simulink model "ComplexPhaseDetectorDual"  (R2016a)
settings: Solver=VariableStepAuto  StartTime=0.0  StopTime=.05  RelTol=1e-6
PreLoadFcn:
  | Bits = 4
  | Ts=2*3/280e6
  | dBRange=11
  | maxNumErrs=500
  | maxNumBits=1e6
  | AM_Gain=AM_GainDiff;
  | AGC_Gain=AGC_GainCalc;
  | load('IIR_Coeffs.mat');
InitFcn:
  | Br= 1/(10*Ts)
  | FreqOffset=00
  | Mode=2
  | BitsPer=[2,2,1,1]
  | EbNo=50
  | N=6
undefined symbols (not defined in the file or in its folder): designMultirateFIR, DiscIntNeverNeededParam
libraries: xbsIndex_r4 x1085, commfilt2 x12, commsink2 x6, dspsigops x5, dspmlti4 x2, commrfcorlib x2, commchan3 x2, dspfdesign x2, dspstat3 x2, commdigbbndpm3 x1, commrandsrc3 x1
(part 1 of 13)
settings Model: Creator=frank.ziegler  LastModifiedBy=frank
settings DebuggingCC: ConsistencyChecking=warning  ArrayBoundsChecking=error  UniqueDataStoreMsg=error

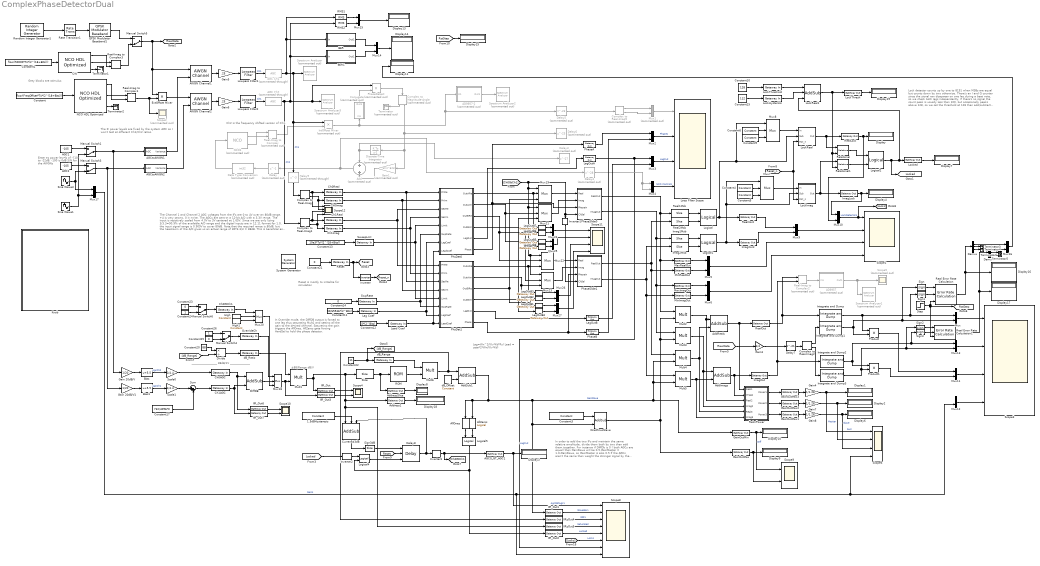
== system ComplexPhaseDetectorDual ==
  note: Lag=Wn^2/(Kv*Kd*Fs)
      | Lead = zeta*2*Wn/(Kv*Kd)
  note: Lock detector counts up by one to 8191 when MSBs are equal but counts down by two otherwise. There's an I and Q counter since the signal can disappear on one leg during a beat note, so we check both legs independently. If there's no signal the count peak is usually less than 100, but occasionally peaks above 128, so we set the threshold at 128 then add/subtract 112 of hysterisis such that both signals have to drop below 16 to loose lock, then either rise above 240. This gives a strong confidence to the lock and allows the 8192 a long time (76uS) to count down to 256 during a fade.
      | Note, the higher the beat note in the IF, the more false negative at high noise levels. At 800Hz I've seen an error every 10 seconds or so.
  note: Reset is mostly to initialize for simulation
  note: Enter as power levels of -110 to -22dB.
      | -100 is 0dB S/N for the AWGNs
  note: The IF power levels are fixed by the system AGC so I won't test at different Ch1/Ch2 ratios.
  note: Ch2 is the frequency shifted version of Ch1.
  note: The Channel 1 and Channel 2 AGC voltages from the IFs are 0 to 4V over an 80dB range. +4 is very strong, 0 is noise. The AGCs are sent to a 12-bit A/D with a 3.3V range. The input is resistively scaled from 4.0V to 3V centered at 1.65V. Since we are only using 3/3.3=90.9% of the available A/D range and the digital inputs are in 12.11 format for 1.0, the input signal range is 0.909V to cover 80dB.
      | Note that the required range is 80dB, but the headroom of the A/D gives us an actual range of 80*3.3/3 = 88dB. This is beneficial as shown below.
      | We take the difference in AGC voltage between the two channels to define the weighting system based on the stronger signal. If we take the differential and multiply by 8 with saturation this effectively gives us a ± 11dB differential maximum. We can use this to limit the range the combiner attempts to work over since combining is only useful over a 10dB range. The nature of the saturation forces a "Best Source Select" function automatically. We take the sign to define the larger channel. The value addresses a look up table that does the log to linear conversion over a 16384-bit resolution. The Log2Lin transposes the log nature of the AGC to a linear ratio of the two signals. If the two AGCs are the same, the differential is zero and the weights are set to 50-50 for optimal combining. As the difference approaches +1.0, the largest signal gets a weight of 100%.and the other is shut off with a weight of 0%.
  note: Grey blocks are stimulus
  note: In order to add the two IFs and maintain the same relative amplitude, divide them both by two then add them together.
      | For instance if DiffDb is 0 ( both AGCs are equal) then GainSlave will be 0.5.GainMaster = 1.0-GainSlave, so GainMaster is also 0.5
      | If the AGCs aren't the same then weight the stronger signal by the differential.
      | If  GainSlave saturates, ignore the lock and pick the larger signal immediately
  note: In Override mode, the DiffDB output is forced to one leg thus saturating Mult1 and setting all the gain to the desired channel. Saturating the gain triggers the AllOnes, AllZeros gate forcing HardSel to hold the phase detector.
  note: ±88/Range dB/V
  note: ___________________ 88dB/1V _______________
  " System Generator" : xbsIndex_r4/ System Generator  Tag=genX  xilinxfamily=kintex7  part=xc7k325t  speed=-2  package=fbg676  synthesis_tool=Vivado  clock_wrapper=Clock Enables  directory=./netlist  proj_type=Vivado  Synth_file=Vivado Synthesis Defaults  Impl_file=Vivado Implementation Defaults  testbench=off  simulink_period=Ts  sysclk_period=2*3000/280  dcm_input_clock_period=10  incr_netlist=off  trim_vbits=Everywhere in SubSystem  dbl_ovrd=According to Block Masks  core_generation=According to Block Masks  run_coregen=off  deprecated_control=off  eval_field=0  block_type=sysgen
  1.5dBHysteresis : xbsIndex_r4/Constant  const=1.5/11  gui_display_data_type=Fixed-point  arith_type=Signed (2's comp)  n_bits=18  bin_pt=17  preci_type=Single  exp_width=8  frac_width=24  explicit_period=on  period=Ts  equ=P=C  opselect=C  inp2=PCIN>>17  opr=+  inp1=P  carry=CIN  dbl_ovrd=off  block_type=constant
  AD9957 : Subsystem  Commented=on
  AD9957-2 : Subsystem  Commented=on
  AGC Ch1 : commrfcorlib/AGC  Commented=through  LegacyMode=off  DetectorMethod=Rectifier  LoopMethod=Linear  UpdatePeriod=100  StepSize=0.1  AdaptationStepSize=0.001  DesiredOutputPower=.05  AveragingLength=100  MaximumGain=30  MaxPowerGain=6  GainOutputPort=off  InputPowerOutputPort=off  SimulateUsing=Interpreted execution
  AGC Ch2 : commrfcorlib/AGC  Commented=through  LegacyMode=off  DetectorMethod=Rectifier  LoopMethod=Linear  UpdatePeriod=100  StepSize=0.1  AdaptationStepSize=0.001  DesiredOutputPower=.05  AveragingLength=100  MaximumGain=30  MaxPowerGain=6  GainOutputPort=off  InputPowerOutputPort=off  SimulateUsing=Interpreted execution
  AGC0_GT_AGC1 : xbsIndex_r4/Gateway Out  inherit_from_input=off  hdl_port=on  rows=1  columns=1  UseAsDAC=off  DACChannel='1'  interface=None  automatic_assignment=on  address_offset=hex2dec('00')  intf_name=''  intf_description=''  timing_constraint=None  locs_specified=off  LOCs={}  io_standard={}  block_type=gatewayout
  AGC1 : Constant  Value=-105  OutDataTypeStr=double
  AGC2 : Constant  Value=-105  OutDataTypeStr=double
  AGCtoAWGN1 : Subsystem
  AGCtoAWGN2 : Subsystem
  AWGN Channel1 : commchan3/AWGN Channel  InputProcessing=Columns as channels (frame based)  seed=67  noiseMode=Variance from port  EbNodB=4  EsNodB=10  SNRdB=10  bitsPerSym=BitsPer(Mode)  Ps=0.707  Tsym=1/Br  variance=1
  AWGN Channel2 : commchan3/AWGN Channel  InputProcessing=Columns as channels (frame based)  seed=70  noiseMode=Variance from port  EbNodB=6  EsNodB=10  SNRdB=10  bitsPerSym=BitsPer(Mode)  Ps=0.707  Tsym=1/Br  variance=1
  Add : Sum  Commented=on  OutDataTypeStr=Inherit: Same as first input
  AddImags : xbsIndex_r4/AddSub  mode=Addition  use_carryin=off  use_carryout=off  en=off  latency=1  precision=User Defined  arith_type="Signed  (2's comp)"  n_bits=18  bin_pt=17  quantization="Round  (unbiased: +/- Inf)"  overflow=Saturate  use_behavioral_HDL=off  hw_selection=Fabric  pipelined=off  dbl_ovrd=off  block_type=addsub
  AddReals : xbsIndex_r4/AddSub  mode=Addition  use_carryin=off  use_carryout=off  en=off  latency=1  precision=User Defined  arith_type="Signed  (2's comp)"  n_bits=18  bin_pt=17  quantization="Round  (unbiased: +/- Inf)"  overflow=Saturate  use_behavioral_HDL=off  hw_selection=Fabric  pipelined=off  dbl_ovrd=off  block_type=addsub
  AddSub1 : xbsIndex_r4/AddSub  mode=Addition  use_carryin=off  use_carryout=off  en=off  latency=1  precision=User Defined  arith_type=Unsigned  n_bits=18  bin_pt=18  quantization=Truncate  overflow=Saturate  use_behavioral_HDL=off  hw_selection=Fabric  pipelined=off  dbl_ovrd=off  block_type=addsub
  Address1 : xbsIndex_r4/Gateway Out  inherit_from_input=off  hdl_port=off  rows=1  columns=1  UseAsDAC=off  DACChannel='1'  interface=None  automatic_assignment=on  address_offset=hex2dec('00')  intf_name=''  intf_description=''  timing_constraint=None  locs_specified=off  LOCs={}  io_standard={}  block_type=gatewayout
  AddressSlice : xbsIndex_r4/Gateway Out  inherit_from_input=off  hdl_port=off  rows=1  columns=1  UseAsDAC=off  DACChannel='1'  interface=None  automatic_assignment=on  address_offset=hex2dec('00')  intf_name=''  intf_description=''  timing_constraint=None  locs_specified=off  LOCs={}  io_standard={}  block_type=gatewayout
  AllOnes : xbsIndex_r4/Logical  logical_function=AND  inputs=1  en=off  latency=0  precision=Full  arith_type=Unsigned  n_bits=16  bin_pt=0  align_bp=on  dbl_ovrd=off  block_type=logical
  AllZeros : xbsIndex_r4/Logical  logical_function=NOR  inputs=1  en=off  latency=0  precision=Full  arith_type=Unsigned  n_bits=16  bin_pt=0  align_bp=on  dbl_ovrd=off  block_type=logical
  BER : Subsystem
  BER1 : Subsystem
  Bias : Bias  Bias=5.5
  Bias1 : Bias  Bias=5.5
  CW : dspsigops/NCO HDL Optimized  PhaseIncrementSource=Input port  PhaseIncrement=100  PhaseOffsetSource=Property  PhaseOffset=0  DitherSource=Property  NumDitherBits=4  PhaseQuantization=on  NumQuantizerAccumulatorBits=12  LUTCompress=off  ResetAction=off  ValidInputPort=off  Waveform=Sine and cosine  PhasePort=off  AccumulatorWL=18+Bits  OutputDataType=double  OutputWL=16  OutputFL=14  SimulateUsing=Code generation
  Ch0AGC : xbsIndex_r4/Gateway In  gui_display_data_type=Fixed-point  arith_type=Unsigned  n_bits=13  bin_pt=12  preci_type=Single  exp_width=8  frac_width=24  rows=1  columns=1  quantization="Round  (unbiased: +/- Inf)"  overflow=Saturate  period=Ts  UseAsADC=off  ADCChannel='1'  interface=None  automatic_assignment=on  address_offset=hex2dec('00')  intf_name=''  intf_description=''  default_value=0  timing_constraint=None  locs_specified=off  LOCs={}  io_standard={}  inherit_from_input=off  hdl_port=on  dbl_ovrd=off  block_type=gatewayin
  Ch0GtCh1 : xbsIndex_r4/Gateway In  gui_display_data_type=Boolean  arith_type=Boolean  n_bits=18  bin_pt=9  preci_type=Single  exp_width=8  frac_width=24  rows=1  columns=1  quantization="Round  (unbiased: +/- Inf)"  overflow=Wrap  period=Ts  UseAsADC=off  ADCChannel='1'  interface=None  automatic_assignment=on  address_offset=hex2dec('00')  intf_name='axi4'  intf_description='Lead Coefficient'  default_value=10  timing_constraint=None  locs_specified=off  LOCs={}  io_standard={}  inherit_from_input=off  hdl_port=on  dbl_ovrd=off  block_type=gatewayin
  Ch0Imag : xbsIndex_r4/Gateway In  gui_display_data_type=Fixed-point  arith_type="Signed  (2's comp)"  n_bits=18  bin_pt=17  preci_type=Single  exp_width=8  frac_width=24  rows=1  columns=1  quantization="Round  (unbiased: +/- Inf)"  overflow=Saturate  period=Ts  UseAsADC=off  ADCChannel='1'  interface=None  automatic_assignment=on  address_offset=hex2dec('00')  intf_name=''  intf_description=''  default_value=0  timing_constraint=None  locs_specified=off  LOCs={}  io_standard={}  inherit_from_input=off  hdl_port=on  dbl_ovrd=off  block_type=gatewayin
  Ch0Real : xbsIndex_r4/Gateway In  gui_display_data_type=Fixed-point  arith_type="Signed  (2's comp)"  n_bits=18  bin_pt=17  preci_type=Single  exp_width=8  frac_width=24  rows=1  columns=1  quantization="Round  (unbiased: +/- Inf)"  overflow=Saturate  period=Ts  UseAsADC=off  ADCChannel='1'  interface=None  automatic_assignment=on  address_offset=hex2dec('00')  intf_name=''  intf_description=''  default_value=0  timing_constraint=None  locs_specified=off  LOCs={}  io_standard={}  inherit_from_input=off  hdl_port=on  dbl_ovrd=off  block_type=gatewayin
  Ch1AGC : xbsIndex_r4/Gateway In  gui_display_data_type=Fixed-point  arith_type=Unsigned  n_bits=13  bin_pt=12  preci_type=Single  exp_width=8  frac_width=24  rows=1  columns=1  quantization="Round  (unbiased: +/- Inf)"  overflow=Saturate  period=Ts  UseAsADC=off  ADCChannel='1'  interface=None  automatic_assignment=on  address_offset=hex2dec('00')  intf_name=''  intf_description=''  default_value=0  timing_constraint=None  locs_specified=off  LOCs={}  io_standard={}  inherit_from_input=off  hdl_port=on  dbl_ovrd=off  block_type=gatewayin
  Ch1Imag : xbsIndex_r4/Gateway In  gui_display_data_type=Fixed-point  arith_type="Signed  (2's comp)"  n_bits=18  bin_pt=17  preci_type=Single  exp_width=8  frac_width=24  rows=1  columns=1  quantization="Round  (unbiased: +/- Inf)"  overflow=Saturate  period=Ts  UseAsADC=off  ADCChannel='1'  interface=None  automatic_assignment=on  address_offset=hex2dec('00')  intf_name=''  intf_description=''  default_value=0  timing_constraint=None  locs_specified=off  LOCs={}  io_standard={}  inherit_from_input=off  hdl_port=on  dbl_ovrd=off  block_type=gatewayin
  Ch1Real : xbsIndex_r4/Gateway In  gui_display_data_type=Fixed-point  arith_type="Signed  (2's comp)"  n_bits=18  bin_pt=17  preci_type=Single  exp_width=8  frac_width=24  rows=1  columns=1  quantization="Round  (unbiased: +/- Inf)"  overflow=Saturate  period=Ts  UseAsADC=off  ADCChannel='1'  interface=None  automatic_assignment=on  address_offset=hex2dec('00')  intf_name=''  intf_description=''  default_value=0  timing_constraint=None  locs_specified=off  LOCs={}  io_standard={}  inherit_from_input=off  hdl_port=on  dbl_ovrd=off  block_type=gatewayin
  Complex to Magnitude-Angle : ComplexToMagnitudeAngle  Commented=on
  Complex to Real-Imag : ComplexToRealImag
  Complex to Real-Imag1 : ComplexToRealImag
  Complex to Real-Imag2 : ComplexToRealImag
  Complex to Real-Imag5 : ComplexToRealImag  Commented=on
  Conjugate : Subsystem  Commented=on
  Constant : Constant  Value=floor(FreqOffset*Ts*(2^(18+Bits)))  OutDataTypeStr=int32  SampleTime=Ts
  Constant1 : Constant  Value=floor(50000*Ts*(2^(18+Bits)))  OutDataTypeStr=int32  SampleTime=Ts
  Constant10 : Constant  Value=128
  Constant11 : Constant  Value=50/65536*(2^Bits)  OutDataTypeStr=double
  Constant12 : Constant  Value=5*(2^Bits)  OutDataTypeStr=double
  Constant13 : Constant  Value=10e3*Ts*(2^(18+Bits))  OutDataTypeStr=double
  Constant{14,21,23,25} (4 alike) : Constant  Value=0  OutDataTypeStr=double
  Constant15 : Constant  Value=112
  Constant17 : Constant  Value=732/4096*0
  Constant20 : Constant  Value=88  OutDataTypeStr=double
  Constant22 : Constant  Value=11  OutDataTypeStr=double
  Constant24 : Constant  OutDataTypeStr=double
  Constant26 : Constant  OutDataTypeStr=double
  Constant3 : xbsIndex_r4/Constant  const=1.0  gui_display_data_type=Fixed-point  arith_type=Unsigned  n_bits=18  bin_pt=18  preci_type=Single  exp_width=8  frac_width=24  explicit_period=on  period=Ts  equ=P=C  opselect=C  inp2=PCIN>>17  opr=+  inp1=P  carry=CIN  dbl_ovrd=off  block_type=constant
  Constant4 : xbsIndex_r4/Constant  const=1  gui_display_data_type=Fixed-point  arith_type=Unsigned  n_bits=8  bin_pt=0  preci_type=Single  exp_width=8  frac_width=24  explicit_period=off  period=1  equ=P=C  opselect=C  inp2=PCIN>>17  opr=+  inp1=P  carry=CIN  dbl_ovrd=off  block_type=constant
  Constant5 : xbsIndex_r4/Constant  const=2  gui_display_data_type=Fixed-point  arith_type=Unsigned  n_bits=8  bin_pt=0  preci_type=Single  exp_width=8  frac_width=24  explicit_period=off  period=1  equ=P=C  opselect=C  inp2=PCIN>>17  opr=+  inp1=P  carry=CIN  dbl_ovrd=off  block_type=constant
  Constant6 : xbsIndex_r4/Constant  const=1  gui_display_data_type=Fixed-point  arith_type=Unsigned  n_bits=8  bin_pt=0  preci_type=Single  exp_width=8  frac_width=24  explicit_period=off  period=1  equ=P=C  opselect=C  inp2=PCIN>>17  opr=+  inp1=P  carry=CIN  dbl_ovrd=off  block_type=constant
  Constant9 : xbsIndex_r4/Constant  const=2  gui_display_data_type=Fixed-point  arith_type=Unsigned  n_bits=8  bin_pt=0  preci_type=Single  exp_width=8  frac_width=24  explicit_period=off  period=1  equ=P=C  opselect=C  inp2=PCIN>>17  opr=+  inp1=P  carry=CIN  dbl_ovrd=off  block_type=constant
  Current±3dB : xbsIndex_r4/AddSub  mode=Addition or Subtraction  use_carryin=off  use_carryout=off  en=off  latency=0  precision=User Defined  arith_type="Signed  (2's comp)"  n_bits=12  bin_pt=11  quantization=Truncate  overflow=Saturate  use_behavioral_HDL=off  hw_selection=Fabric  pipelined=off  dbl_ovrd=off  block_type=addsub
  Data Type Conversion : DataTypeConversion  Commented=on  OutDataTypeStr=int32  SaturateOnIntegerOverflow=on
  Delay : Delay  Commented=on  DelayLength=1
  Delay3 : Delay  Commented=on  DelayLength=27
  Delay4 : Delay  Commented=on  DelayLength=28
  Delay5 : Delay  Commented=on  DelayLength=23
  Delay6 : Delay  Commented=on  DelayLength=23
  Delay7 : Delay  DelayLength=21
  Delay8 : xbsIndex_r4/Delay  rst=on  infoeditControl=Selection of Reset will increase slice count due to use of real FFs and instead of SRLs  en=on  latency=1  reg_retiming=off  dbl_ovrd=off  block_type=delay
  Delay9 : Delay  Commented=through  DelayLength=3
  Demux : Demux  Outputs=3
  Demux1 : Demux  Outputs=3
  DiffDB : xbsIndex_r4/AddSub  mode=Subtraction  use_carryin=off  use_carryout=off  en=off  latency=1  precision=Full  arith_type="Signed  (2's comp)"  n_bits=13  bin_pt=12  quantization=Truncate  overflow=Saturate  use_behavioral_HDL=off  hw_selection=Fabric  pipelined=off  dbl_ovrd=off  block_type=addsub
  Discrete-Time Integrator : DiscreteIntegrator  Commented=on  gainval=(2^Bits)*50/65536/Ts  InitialConditionSetting=State (most efficient)  SampleTime=Ts  ICPrevOutput=DiscIntNeverNeededParam  ICPrevScaledInput=DiscIntNeverNeededParam
  Display{,1..4,6..11,13..19} (18 alike) : Display
      Display11 settings: Format=short_e
      Display14 settings: Format=short_e
  Divide : Product  Inputs=*/
  ExtOffset Mixer : Product
  Gain 20dB/V : Gain  Gain=1/20
  Gain 20dB/V1 : Gain  Gain=1/20
  Gain1 : Gain  Commented=on  Gain=5*(2^Bits)
  Gain3 : Gain  Gain=1/4
  Gain4 : Gain  Gain=1/1.26
  Gain5 : Gain  Gain=.25
  Gain6 : Gain  Gain=.25
  Gain7 : Gain  Gain=1/1.26
  Gain8 : Gain  Gain=1/1.26
  GainOutMax : xbsIndex_r4/Gateway Out  inherit_from_input=off  hdl_port=on  rows=1  columns=1  UseAsDAC=off  DACChannel='1'  interface=None  automatic_assignment=on  address_offset=hex2dec('00')  intf_name=''  intf_description=''  timing_constraint=None  locs_specified=off  LOCs={}  io_standard={}  block_type=gatewayout
  GainOutMax1 : xbsIndex_r4/Gateway Out  inherit_from_input=off  hdl_port=off  rows=1  columns=1  UseAsDAC=off  DACChannel='1'  interface=None  automatic_assignment=on  address_offset=hex2dec('00')  intf_name=''  intf_description=''  timing_constraint=None  locs_specified=off  LOCs={}  io_standard={}  block_type=gatewayout
  GainOutMax2 : xbsIndex_r4/Gateway Out  inherit_from_input=off  hdl_port=off  rows=1  columns=1  UseAsDAC=off  DACChannel='1'  interface=None  automatic_assignment=on  address_offset=hex2dec('00')  intf_name=''  intf_description=''  timing_constraint=None  locs_specified=off  LOCs={}  io_standard={}  block_type=gatewayout
  GainOutMax3 : xbsIndex_r4/Gateway Out  inherit_from_input=off  hdl_port=off  rows=1  columns=1  UseAsDAC=off  DACChannel='1'  interface=None  automatic_assignment=on  address_offset=hex2dec('00')  intf_name=''  intf_description=''  timing_constraint=None  locs_specified=off  LOCs={}  io_standard={}  block_type=gatewayout
  GainOutMin : xbsIndex_r4/Gateway Out  inherit_from_input=off  hdl_port=on  rows=1  columns=1  UseAsDAC=off  DACChannel='1'  interface=None  automatic_assignment=on  address_offset=hex2dec('00')  intf_name=''  intf_description=''  timing_constraint=None  locs_specified=off  LOCs={}  io_standard={}  block_type=gatewayout
  High : xbsIndex_r4/Constant  const=.75  gui_display_data_type=Fixed-point  arith_type=Signed (2's comp)  n_bits=14  bin_pt=12  preci_type=Single  exp_width=8  frac_width=24  explicit_period=on  period=Ts  equ=P=C  opselect=C  inp2=PCIN>>17  opr=+  inp1=P  carry=CIN  dbl_ovrd=off  block_type=constant
  High1 : xbsIndex_r4/Constant  const=-.75  gui_display_data_type=Fixed-point  arith_type=Signed (2's comp)  n_bits=14  bin_pt=12  preci_type=Single  exp_width=8  frac_width=24  explicit_period=on  period=Ts  equ=P=C  opselect=C  inp2=PCIN>>17  opr=+  inp1=P  carry=CIN  dbl_ovrd=off  block_type=constant
  IIR_Out{,1..7} (8 alike) : xbsIndex_r4/Gateway Out  inherit_from_input=off  hdl_port=off  rows=1  columns=1  UseAsDAC=off  DACChannel='1'  interface=None  automatic_assignment=on  address_offset=hex2dec('00')  intf_name=''  intf_description=''  timing_constraint=None  locs_specified=off  LOCs={}  io_standard={}  block_type=gatewayout
  Imag1Msb : xbsIndex_r4/Slice  nbits=1  boolean_output=on  mode=Upper Bit Location + Width  bit1=0  base1=MSB of Input  bit0=0  base0=LSB of Input  dbl_ovrd=off  block_type=slice
  Imag2Msb : xbsIndex_r4/Slice  nbits=1  boolean_output=on  mode=Upper Bit Location + Width  bit1=0  base1=MSB of Input  bit0=0  base0=LSB of Input  dbl_ovrd=off  block_type=slice
  ImagLock : xbsIndex_r4/Gateway Out  inherit_from_input=off  hdl_port=on  rows=1  columns=1  UseAsDAC=off  DACChannel='1'  interface=None  automatic_assignment=on  address_offset=hex2dec('00')  intf_name=''  intf_description=''  timing_constraint=None  locs_specified=off  LOCs={}  io_standard={}  block_type=gatewayout
  ImagOut : xbsIndex_r4/Gateway Out  inherit_from_input=off  hdl_port=on  rows=1  columns=1  UseAsDAC=off  DACChannel='1'  interface=None  automatic_assignment=on  address_offset=hex2dec('00')  intf_name=''  intf_description=''  timing_constraint=None  locs_specified=off  LOCs={}  io_standard={}  block_type=gatewayout
  ImagXord : xbsIndex_r4/Gateway Out  inherit_from_input=off  hdl_port=on  rows=1  columns=1  UseAsDAC=off  DACChannel='1'  interface=None  automatic_assignment=on  address_offset=hex2dec('00')  intf_name=''  intf_description=''  timing_constraint=None  locs_specified=off  LOCs={}  io_standard={}  block_type=gatewayout
  IntOffset Mixer : Product  Commented=on
  Integrate and Dump{,1..3} (4 alike) : commfilt2/Integrate and Dump  obssamples=10  offsetsamples=2  nodump=off  roundingMode=Floor  overflowMode=off  outputDataTypeStr=Inherit: Same as accumulator  outputLastDataTypeStr=Inherit: Same as accumulator
  Inverter{,1..3} (4 alike) : xbsIndex_r4/Inverter  en=off  latency=0  dbl_ovrd=off  block_type=inv
  Knob : Subsystem  DialogController=hmiCreateDDGDialog  IsWebBlock=on  mask(MWDashboardBlock){webBlockId=e460d0c1-8f1d-4963-a065-60dc3f9fc9ee, webBlockType=continuousknob, ShowInLibBrowser=on, ShowInitialText=on, HMISrcModelName=ComplexPhaseDetectorDual}
      mask prompts: webBlockId "WebBlock Id"; webBlockType "WebBlock Type"; HMISrcModelName "Source Model"
      mask Help: helpview([docroot '/mapfiles/simulink.map'], 'hmi_knob')
      mask Display:
      | if strcmp(get_param(bdroot(gcb),'BlockDiagramType'), 'library')
      |     image([(matlabroot) '/toolbox/simulink/hmi/icons/ContinuousKnob.png']);
      | end
  Lag Coef : xbsIndex_r4/Gateway In  gui_display_data_type=Fixed-point  arith_type=Unsigned  n_bits=18  bin_pt=17  preci_type=Single  exp_width=8  frac_width=24  rows=1  columns=1  quantization="Round  (unbiased: +/- Inf)"  overflow=Wrap  period=Ts  UseAsADC=off  ADCChannel='1'  interface=None  automatic_assignment=on  address_offset=hex2dec('00')  intf_name='axi4'  intf_description='Lead Coefficient'  default_value=5*Ts  timing_constraint=None  locs_specified=off  LOCs={}  io_standard={}  inherit_from_input=off  hdl_port=on  dbl_ovrd=off  block_type=gatewayin
  LagOutA : xbsIndex_r4/Gateway Out  inherit_from_input=off  hdl_port=on  rows=1  columns=1  UseAsDAC=off  DACChannel='1'  interface=None  automatic_assignment=on  address_offset=hex2dec('00')  intf_name=''  intf_description=''  timing_constraint=None  locs_specified=off  LOCs={}  io_standard={}  block_type=gatewayout
  LagOutB : xbsIndex_r4/Gateway Out  inherit_from_input=off  hdl_port=on  rows=1  columns=1  UseAsDAC=off  DACChannel='1'  interface=None  automatic_assignment=on  address_offset=hex2dec('00')  intf_name=''  intf_description=''  timing_constraint=None  locs_specified=off  LOCs={}  io_standard={}  block_type=gatewayout
  LagOutB{1..8} (8 alike) : xbsIndex_r4/Gateway Out  inherit_from_input=off  hdl_port=off  rows=1  columns=1  UseAsDAC=off  DACChannel='1'  interface=None  automatic_assignment=on  address_offset=hex2dec('00')  intf_name=''  intf_description=''  timing_constraint=None  locs_specified=off  LOCs={}  io_standard={}  block_type=gatewayout
  Lead Coef : xbsIndex_r4/Gateway In  gui_display_data_type=Fixed-point  arith_type=Unsigned  n_bits=18  bin_pt=9  preci_type=Single  exp_width=8  frac_width=24  rows=1  columns=1  quantization="Round  (unbiased: +/- Inf)"  overflow=Wrap  period=Ts  UseAsADC=off  ADCChannel='1'  interface=None  automatic_assignment=on  address_offset=hex2dec('00')  intf_name='axi4'  intf_description='Lead Coefficient'  default_value=10  timing_constraint=None  locs_specified=off  LOCs={}  io_standard={}  inherit_from_input=off  hdl_port=on  dbl_ovrd=off  block_type=gatewayin
  LockHysterisis : xbsIndex_r4/Gateway In  gui_display_data_type=Fixed-point  arith_type=Unsigned  n_bits=13  bin_pt=0  preci_type=Single  exp_width=8  frac_width=24  rows=1  columns=1  quantization="Round  (unbiased: +/- Inf)"  overflow=Wrap  period=Ts  UseAsADC=off  ADCChannel='1'  interface=None  automatic_assignment=on  address_offset=hex2dec('00')  intf_name=''  intf_description=''  default_value=0  timing_constraint=None  locs_specified=off  LOCs={}  io_standard={}  inherit_from_input=off  hdl_port=on  dbl_ovrd=off  block_type=gatewayin
  LockImag : Subsystem
  LockReal : Subsystem
  LockReal1 : xbsIndex_r4/AddSub  mode=Addition or Subtraction  use_carryin=off  use_carryout=off  en=off  latency=0  precision=User Defined  arith_type=Unsigned  n_bits=13  bin_pt=0  quantization=Truncate  overflow=Wrap  use_behavioral_HDL=off  hw_selection=Fabric  pipelined=off  dbl_ovrd=off  block_type=addsub
  LockThresh : xbsIndex_r4/Gateway Out  inherit_from_input=off  hdl_port=off  rows=1  columns=1  UseAsDAC=off  DACChannel='1'  interface=None  automatic_assignment=on  address_offset=hex2dec('00')  intf_name=''  intf_description=''  timing_constraint=None  locs_specified=off  LOCs={}  io_standard={}  block_type=gatewayout
  LockThreshold : xbsIndex_r4/Gateway In  gui_display_data_type=Fixed-point  arith_type=Unsigned  n_bits=13  bin_pt=0  preci_type=Single  exp_width=8  frac_width=24  rows=1  columns=1  quantization="Round  (unbiased: +/- Inf)"  overflow=Wrap  period=Ts  UseAsADC=off  ADCChannel='1'  interface=None  automatic_assignment=on  address_offset=hex2dec('00')  intf_name=''  intf_description=''  default_value=0  timing_constraint=None  locs_specified=off  LOCs={}  io_standard={}  inherit_from_input=off  hdl_port=on  dbl_ovrd=off  block_type=gatewayin
  Locked : xbsIndex_r4/Gateway Out  inherit_from_input=off  hdl_port=on  rows=1  columns=1  UseAsDAC=off  DACChannel='1'  interface=None  automatic_assignment=on  address_offset=hex2dec('00')  intf_name=''  intf_description=''  timing_constraint=None  locs_specified=off  LOCs={}  io_standard={}  block_type=gatewayout
  Logical : xbsIndex_r4/Logical  logical_function=XOR  inputs=2  en=off  latency=1  precision=Full  arith_type=Unsigned  n_bits=16  bin_pt=0  align_bp=on  dbl_ovrd=off  block_type=logical
  Logical1 : xbsIndex_r4/Logical  logical_function=XOR  inputs=2  en=off  latency=1  precision=Full  arith_type=Unsigned  n_bits=16  bin_pt=0  align_bp=on  dbl_ovrd=off  block_type=logical
  Logical2 : xbsIndex_r4/Logical  logical_function=OR  inputs=2  en=off  latency=1  precision=Full  arith_type=Boolean  n_bits=16  bin_pt=0  align_bp=on  dbl_ovrd=off  block_type=logical
  Logical4 : xbsIndex_r4/Logical  logical_function=OR  inputs=2  en=off  latency=0  precision=Full  arith_type=Unsigned  n_bits=16  bin_pt=0  align_bp=on  dbl_ovrd=off  block_type=logical
  Logical5 : xbsIndex_r4/Logical  logical_function=OR  inputs=2  en=off  latency=0  precision=Full  arith_type=Unsigned  n_bits=16  bin_pt=0  align_bp=on  dbl_ovrd=off  block_type=logical
  Loop Filter Scope : Scope  NumInputPorts=4
  Lowpass Filter1 : dspfdesign/Lowpass Filter  FilterType=FIR  DesignForMinimumOrder=off  FilterOrder=26  PassbandFrequency=Br/2  StopbandFrequency=Br*2  PassbandRipple=0.1  StopbandAttenuation=80  InheritSampleRate=off  SampleRate=1/Ts  roundingMode=Floor  coeffsDataTypeStr=fixdt(1,16)  SimulateUsing=Interpreted execution
  Lowpass Filter2 : dspfdesign/Lowpass Filter  FilterType=FIR  DesignForMinimumOrder=off  FilterOrder=26  PassbandFrequency=Br/2  StopbandFrequency=Br*2  PassbandRipple=0.1  StopbandAttenuation=80  InheritSampleRate=off  SampleRate=1/Ts  roundingMode=Floor  coeffsDataTypeStr=fixdt(1,16)  SimulateUsing=Interpreted execution
  Manual Switch{1,3..6} (5 alike) : ManualSwitch  CurrentSetting=0
  MaxImagOut : xbsIndex_r4/Gateway Out  inherit_from_input=off  hdl_port=on  rows=1  columns=1  UseAsDAC=off  DACChannel='1'  interface=None  automatic_assignment=on  address_offset=hex2dec('00')  intf_name=''  intf_description=''  timing_constraint=None  locs_specified=off  LOCs={}  io_standard={}  block_type=gatewayout
  MaxRealOut : xbsIndex_r4/Gateway Out  inherit_from_input=off  hdl_port=on  rows=1  columns=1  UseAsDAC=off  DACChannel='1'  interface=None  automatic_assignment=on  address_offset=hex2dec('00')  intf_name=''  intf_description=''  timing_constraint=None  locs_specified=off  LOCs={}  io_standard={}  block_type=gatewayout
  MinImagOut : xbsIndex_r4/Gateway Out  inherit_from_input=off  hdl_port=on  rows=1  columns=1  UseAsDAC=off  DACChannel='1'  interface=None  automatic_assignment=on  address_offset=hex2dec('00')  intf_name=''  intf_description=''  timing_constraint=None  locs_specified=off  LOCs={}  io_standard={}  block_type=gatewayout
  MinRealOut : xbsIndex_r4/Gateway Out  inherit_from_input=off  hdl_port=on  rows=1  columns=1  UseAsDAC=off  DACChannel='1'  interface=None  automatic_assignment=on  address_offset=hex2dec('00')  intf_name=''  intf_description=''  timing_constraint=None  locs_specified=off  LOCs={}  io_standard={}  block_type=gatewayout
  Mult1 : xbsIndex_r4/Mult  precision=User Defined  arith_type="Signed  (2's comp)"  n_bits=18  bin_pt=17  quantization=Truncate  overflow=Saturate  en=off  latency=3  use_behavioral_HDL=off  opt=Speed  use_embedded=on  optimum_pipeline=off  pipeline=on  dbl_ovrd=off  use_rpm=on  placement_style=Triangular  block_type=mult
  Mult{2..5} (4 alike) : xbsIndex_r4/Mult  precision=User Defined  arith_type="Signed  (2's comp)"  n_bits=18  bin_pt=17  quantization="Round  (unbiased: +/- Inf)"  overflow=Flag as error  en=off  latency=3  use_behavioral_HDL=off  opt=Speed  use_embedded=on  optimum_pipeline=off  pipeline=on  dbl_ovrd=off  use_rpm=on  placement_style=Triangular  block_type=mult
  Mult6 : xbsIndex_r4/Mult  precision=User Defined  arith_type="Signed  (2's comp)"  n_bits=18  bin_pt=17  quantization=Truncate  overflow=Saturate  en=off  latency=3  use_behavioral_HDL=off  opt=Speed  use_embedded=on  optimum_pipeline=off  pipeline=on  dbl_ovrd=off  use_rpm=on  placement_style=Triangular  block_type=mult
  Mux{,2..6,9..17,24..27} (19 alike) : Mux  Inputs=2
  Mux1 : Mux  Commented=on  Inputs=2
  Mux{7..8,18..23} (8 alike) : xbsIndex_r4/Mux  inputs=2  en=off  latency=0  precision=Full  arith_type=Unsigned  n_bits=16  bin_pt=14  quantization=Truncate  overflow=Wrap  dbl_ovrd=off  block_type=mux
  NCO HDL Optimized : dspsigops/NCO HDL Optimized  PhaseIncrementSource=Input port  PhaseIncrement=100  PhaseOffsetSource=Property  PhaseOffset=2^(18+Bits)/8  DitherSource=Property  NumDitherBits=4  PhaseQuantization=on  NumQuantizerAccumulatorBits=12  LUTCompress=off  ResetAction=off  ValidInputPort=off  Waveform=Sine and cosine  PhasePort=off  AccumulatorWL=18+Bits  OutputDataType=double  OutputWL=16  OutputFL=14  SimulateUsing=Code generation
  NCO1 : dspsigops/NCO  Commented=on  AccIncSrc=Input port  AccInc=100  PhaseOffsetSrc=Specify via dialog  PhaseOffset=0  AccumWL=18+Bits  HasDither=off  DitherWL=4  PNgeneratorLength=19  HasPhaseQuantizer=off  TableDepth=12  HasOutputPhaseError=off  Formula=Sine and cosine  DataType=double  OutputWL=16  OutputFL=14  CompMethod=Table lookup (no interpolation)  SampleTime=Ts  SamplesPerFrame=1  OutputFrames=off
  OneMinusSlave : xbsIndex_r4/AddSub  mode=Subtraction  use_carryin=off  use_carryout=off  en=off  latency=0  precision=User Defined  arith_type=Unsigned  n_bits=18  bin_pt=18  quantization=Truncate  overflow=Wrap  use_behavioral_HDL=off  hw_selection=Fabric  pipelined=off  dbl_ovrd=off  block_type=addsub
  OverrideCh : xbsIndex_r4/Gateway In  gui_display_data_type=Boolean  arith_type=Boolean  n_bits=18  bin_pt=9  preci_type=Single  exp_width=8  frac_width=24  rows=1  columns=1  quantization="Round  (unbiased: +/- Inf)"  overflow=Wrap  period=Ts  UseAsADC=off  ADCChannel='1'  interface=None  automatic_assignment=on  address_offset=hex2dec('00')  intf_name='axi4'  intf_description='Lead Coefficient'  default_value=10  timing_constraint=None  locs_specified=off  LOCs={}  io_standard={}  inherit_from_input=off  hdl_port=on  dbl_ovrd=off  block_type=gatewayin
  PhaseA : xbsIndex_r4/Gateway Out  inherit_from_input=off  hdl_port=on  rows=1  columns=1  UseAsDAC=off  DACChannel='1'  interface=None  automatic_assignment=on  address_offset=hex2dec('00')  intf_name=''  intf_description=''  timing_constraint=None  locs_specified=off  LOCs={}  io_standard={}  block_type=gatewayout
  PhaseB : xbsIndex_r4/Gateway Out  inherit_from_input=off  hdl_port=on  rows=1  columns=1  UseAsDAC=off  DACChannel='1'  interface=None  automatic_assignment=on  address_offset=hex2dec('00')  intf_name=''  intf_description=''  timing_constraint=None  locs_specified=off  LOCs={}  io_standard={}  block_type=gatewayout
  PhaseDetect : Product  Commented=on
  PhaseSlide0 : Subsystem
  PhaseSlide1 : Subsystem
  PhsDet0 : Subsystem
  PhsDet1 : Subsystem
  Product : Product
  Product1 : Product
  QPSK Modulator Baseband1 : commdigbbndpm3/QPSK Modulator Baseband  InType=Integer  Enc=Gray  Ph=pi/4  outDtype=double  outWordLen=16  outUDDataType=sfix(16)  outFracLenMode=Best precision  outFracLen=15  outDataTypeStr=double  outLastDataTypeStr=double
  RMS1 : dspstat3/RMS  run=on  reset_popup=None  directionMode=Each column  dimension=1
  RMS2 : dspstat3/RMS  run=on  reset_popup=None  directionMode=Each column  dimension=1
  ROM : xbsIndex_r4/ROM  depth=16384  initVector=AGC_Gain  distributed_mem=Block RAM  rst=off  init_reg=0  en=off  latency=1  gui_display_data_type=Fixed-point  arith_type="Signed  (2's comp)"  n_bits=18  bin_pt=17  preci_type=Single  exp_width=8  frac_width=24  optimize=Area  use_rpm=on  dbl_ovrd=off  block_type=sprom
  Random Integer Generator1 : commrandsrc3/Random Integer Generator  SetSize=4  SeedSource=Auto  Seed=0  SampleTime=1/Br  SamplesPerFrame=1  OutputDataType=double  SimulateUsing=Code generation
  Rate Transition1 : RateTransition  OutPortSampleTime=Ts
  ReImPower : Subsystem
  Real Error Rate Calculation : commsink2/Error Rate Calculation  N=0  st_delay=100  cp_mode=Entire frame  subframe=[]  PMode=Port  WsName=BER  RsMode2=on  stop=off  numErr=maxNumErrs  maxBits=maxNumBits
  Real Error Rate Calculation1 : commsink2/Error Rate Calculation  N=0  st_delay=100  cp_mode=Entire frame  subframe=[]  PMode=Port  WsName=BER  RsMode2=on  stop=off  numErr=maxNumErrs  maxBits=maxNumBits
  Real-Imag to Complex : RealImagToComplex  Commented=on
  Real-Imag to Complex1 : RealImagToComplex
  Real-Imag to Complex2 : RealImagToComplex  Commented=on
  Real-Imag to Complex3 : RealImagToComplex
  Real1Msb : xbsIndex_r4/Slice  nbits=1  boolean_output=on  mode=Upper Bit Location + Width  bit1=0  base1=MSB of Input  bit0=0  base0=LSB of Input  dbl_ovrd=off  block_type=slice
  Real2Msb : xbsIndex_r4/Slice  nbits=1  boolean_output=on  mode=Upper Bit Location + Width  bit1=0  base1=MSB of Input  bit0=0  base0=LSB of Input  dbl_ovrd=off  block_type=slice
  RealLock : xbsIndex_r4/Gateway Out  inherit_from_input=off  hdl_port=on  rows=1  columns=1  UseAsDAC=off  DACChannel='1'  interface=None  automatic_assignment=on  address_offset=hex2dec('00')  intf_name=''  intf_description=''  timing_constraint=None  locs_specified=off  LOCs={}  io_standard={}  block_type=gatewayout
  RealOut : xbsIndex_r4/Gateway Out  inherit_from_input=off  hdl_port=on  rows=1  columns=1  UseAsDAC=off  DACChannel='1'  interface=None  automatic_assignment=on  address_offset=hex2dec('00')  intf_name=''  intf_description=''  timing_constraint=None  locs_specified=off  LOCs={}  io_standard={}  block_type=gatewayout
  RealXord : xbsIndex_r4/Gateway Out  inherit_from_input=off  hdl_port=on  rows=1  columns=1  UseAsDAC=off  DACChannel='1'  interface=None  automatic_assignment=on  address_offset=hex2dec('00')  intf_name=''  intf_description=''  timing_constraint=None  locs_specified=off  LOCs={}  io_standard={}  block_type=gatewayout
  Relational : xbsIndex_r4/Relational  mode=a>=b  op_type=Bool  en=off  latency=0  dbl_ovrd=off  block_type=relational
  Relational1 : xbsIndex_r4/Relational  mode=a>=b  op_type=Bool  en=off  latency=0  dbl_ovrd=off  block_type=relational
  Reset : xbsIndex_r4/Gateway In  gui_display_data_type=Boolean  arith_type=Boolean  n_bits=3  bin_pt=0  preci_type=Single  exp_width=8  frac_width=24  rows=1  columns=1  quantization="Round  (unbiased: +/- Inf)"  overflow=Saturate  period=Ts  UseAsADC=off  ADCChannel='1'  interface=None  automatic_assignment=on  address_offset=hex2dec('00')  intf_name=''  intf_description=''  default_value=0  timing_constraint=None  locs_specified=off  LOCs={}  io_standard={}  inherit_from_input=off  hdl_port=on  dbl_ovrd=off  block_type=gatewayin
  Scale0 : Gain  Gain=1/4.4
  Scale1 : Gain  Gain=1/4.4
  Scope{1,3,6,11..12} (5 alike) : Scope  NumInputPorts=4
  Scope10 : Scope  NumInputPorts=2
  Scope2 : Scope  Commented=on
  Scope4 : Scope  NumInputPorts=2
  Scope5 : Scope  Commented=on
  Scope8 : Scope  NumInputPorts=8
  Scope9 : Scope  NumInputPorts=2
  Sign{,1..3} (4 alike) : Signum
  Sign3dB : xbsIndex_r4/Slice  nbits=1  boolean_output=on  mode=Upper Bit Location + Width  bit1=0  base1=MSB of Input  bit0=0  base0=LSB of Input  dbl_ovrd=off  block_type=slice
  Sine Wave1 : Sin  Amplitude=20  Bias=-50  Frequency=5000*pi()  SampleTime=Ts
  Sine Wave3 : Sin  Amplitude=20  Bias=-50  Frequency=5000*pi()  Phase=pi()  SampleTime=Ts
  Slice : xbsIndex_r4/Slice  nbits=14  boolean_output=off  mode=Upper Bit Location + Width  bit1=0  base1=MSB of Input  bit0=0  base0=LSB of Input  dbl_ovrd=off  block_type=slice
  Spectrum Analyzer{,1..3} (4 alike) : SpectrumAnalyzer  Commented=on
  Step : Step  Time=.0002  Before=1  After=0  SampleTime=1/Br
  Sum : Sum  Inputs=|++
  SweepLmt : xbsIndex_r4/Gateway In  gui_display_data_type=Fixed-point  arith_type=Unsigned  n_bits=11+Bits  bin_pt=0  preci_type=Single  exp_width=8  frac_width=24  rows=1  columns=1  quantization="Round  (unbiased: +/- Inf)"  overflow=Saturate  period=Ts  UseAsADC=off  ADCChannel='1'  interface=None  automatic_assignment=on  address_offset=hex2dec('00')  intf_name='axi4'  intf_description='Lead Coefficient'  default_value=5*Ts  timing_constraint=None  locs_specified=off  LOCs={}  io_standard={}  inherit_from_input=off  hdl_port=on  dbl_ovrd=off  block_type=gatewayin
  SwpRate : xbsIndex_r4/Gateway In  gui_display_data_type=Fixed-point  arith_type="Signed  (2's comp)"  n_bits=18  bin_pt=9  preci_type=Single  exp_width=8  frac_width=24  rows=1  columns=1  quantization="Round  (unbiased: +/- Inf)"  overflow=Wrap  period=Ts  UseAsADC=off  ADCChannel='1'  interface=None  automatic_assignment=on  address_offset=hex2dec('00')  intf_name='axi4'  intf_description='Lead Coefficient'  default_value=5*Ts  timing_constraint=None  locs_specified=off  LOCs={}  io_standard={}  inherit_from_input=off  hdl_port=on  dbl_ovrd=off  block_type=gatewayin
  Terminator : Terminator  Commented=on
  Terminator{1..6} (6 alike) : Terminator
  dB_Offset : xbsIndex_r4/Constant  const=0.5  gui_display_data_type=Fixed-point  arith_type=Signed (2's comp)  n_bits=18  bin_pt=17  preci_type=Single  exp_width=8  frac_width=24  explicit_period=on  period=Ts  equ=P=C  opselect=C  inp2=PCIN>>17  opr=+  inp1=P  carry=CIN  dbl_ovrd=off  block_type=constant
  dB_Range : xbsIndex_r4/Gateway In  gui_display_data_type=Fixed-point  arith_type=Unsigned  n_bits=16  bin_pt=10  preci_type=Single  exp_width=8  frac_width=24  rows=1  columns=1  quantization="Round  (unbiased: +/- Inf)"  overflow=Flag as error  period=Ts  UseAsADC=off  ADCChannel='1'  interface=None  automatic_assignment=on  address_offset=hex2dec('00')  intf_name=''  intf_description=''  default_value=0  timing_constraint=None  locs_specified=off  LOCs={}  io_standard={}  inherit_from_input=off  hdl_port=on  dbl_ovrd=off  block_type=gatewayin
  dB_Ratio : xbsIndex_r4/Gateway In  gui_display_data_type=Fixed-point  arith_type=Unsigned  n_bits=16  bin_pt=6  preci_type=Single  exp_width=8  frac_width=24  rows=1  columns=1  quantization="Round  (unbiased: +/- Inf)"  overflow=Flag as error  period=Ts  UseAsADC=off  ADCChannel='1'  interface=None  automatic_assignment=on  address_offset=hex2dec('00')  intf_name=''  intf_description=''  default_value=0  timing_constraint=None  locs_specified=off  LOCs={}  io_standard={}  inherit_from_input=off  hdl_port=on  dbl_ovrd=off  block_type=gatewayin
  tag scope: Locked=global, RawData=global, Reset=global, Reset_n=global, RstStep=global
  wires:
  Real-Imag to Complex/1 -> IntOffset Mixer/2
  PhaseDetect/1 -> Complex to Magnitude-Angle/1
  Conjugate/1(Out1) -> PhaseDetect/2
  NCO1/2 -> Real-Imag to Complex/1
  NCO1/1 -> Real-Imag to Complex/2
  Discrete-Time Integrator/1 -> Delay3/1, Add/1
  Gain1/1 -> Add/2
  NCO HDL Optimized/1 -> Real-Imag to Complex1/2
  NCO HDL Optimized/2 -> Real-Imag to Complex1/1
  Real-Imag to Complex1/1 -> ExtOffset Mixer/2, Scope2/1
  IntOffset Mixer/1 -> AD9957-2/1(In1), Delay5/1, Conjugate/1(In1)
  Complex to Magnitude-Angle/2 -> Delay6/1, Gain1/1, Discrete-Time Integrator/1
  Complex to Real-Imag/1 -> Scope12/1, Ch0Real/1
  Complex to Real-Imag/2 -> Scope12/2, Ch0Imag/1
  Complex to Real-Imag1/2 -> Scope12/4, Ch1Imag/1
  Complex to Real-Imag1/1 -> Scope12/3, Ch1Real/1
  Complex to Magnitude-Angle/1 -> Terminator/1
  PhaseA/1 -> Mux2/1
  Data Type Conversion/1 -> NCO1/1
  MaxRealOut/1 -> Mux5/1
  MaxImagOut/1 -> Mux6/1
  MinImagOut/1 -> Mux6/2
  MinRealOut/1 -> Mux5/2
  Mux5/1 -> Scope1/3
  Mux6/1 -> Scope1/4
  Bias1/1 -> Scale1/1  "AgcCh1"
  Bias/1 -> Scale0/1  "AgcCh0"
  Mult2/1 -> ReImPower/3(Real2), AddReals/1
  Mult4/1 -> ReImPower/5(Real3), AddReals/2
  Mult5/1 -> ReImPower/6(Imag3), AddImags/2
  Mult3/1 -> ReImPower/4(Imag2), AddImags/1
  AddReals/1 -> ReImPower/1(Real1), RealOut/1
  ImagOut/1 -> Integrate and Dump2/1, Real-Imag to Complex2/2
  AddImags/1 -> ReImPower/2(Imag1), ImagOut/1
  Constant11/1 -> Lag Coef/1
  Constant12/1 -> Lead Coef/1
  AWGN Channel1/1 -> Gain5/1
  Gain5/1 -> Lowpass Filter1/1
  ExtOffset Mixer/1 -> AWGN Channel2/1
  Complex to Real-Imag5/1 -> Mux1/1
  Complex to Real-Imag5/2 -> Mux1/2
  LagOutA/1 -> Scope8/7, Mux3/1  "LagOut"
  Real-Imag to Complex2/1 -> AD9957/1(In1)
  AD9957/1(Out1) -> Scope5/1, Spectrum Analyzer1/1
  Delay5/1 -> Complex to Real-Imag5/1
  AD9957-2/1(Out1) -> Spectrum Analyzer2/1
  Real1Msb/1 -> Logical/1
  Real2Msb/1 -> Logical/2
  RealXord/1 -> Mux9/1
  Imag1Msb/1 -> Logical1/1
  Imag2Msb/1 -> Logical1/2
  ImagXord/1 -> Mux9/2
  RealLock/1 -> Mux10/2, Display/1
  Mux9/1 -> Scope1/2
  Logical1/1 -> LockImag/2(Sub), Mux7/1, ImagXord/1
  LockImag/1(Out) -> Relational1/1, ImagLock/1
  Mux7/1 -> LockImag/1(In)
  ImagLock/1 -> Display4/1, Mux10/1
  Mux10/1 -> [Locks], Scope1/1  "LockDetectors"
  Delay/1 -> Data Type Conversion/1
  Mux3/1 -> Loop Filter Scope/3  "LagOut"
  Mux4/1 -> Loop Filter Scope/4  "NCO Controls"
  Delay4/1 -> Mux4/2, Mux4/1
  Constant4/1 -> Mux7/2
  Constant5/1 -> Mux7/3
  Logical/1 -> LockReal/2(Sub), Mux8/1, RealXord/1
  Constant6/1 -> Mux8/2
  Constant9/1 -> Mux8/3
  Add/1 -> Delay4/1, Delay/1
  Relational1/1 -> Logical2/2
  Relational/1 -> Logical2/1
  Locked/1 -> Display7/1
  Mux2/1 -> Loop Filter Scope/2  "Phases"
  Constant13/1 -> SweepLmt/1
  Constant14/1 -> SwpRate/1
  Delay7/1 -> Complex to Real-Imag2/1
  Product1/1 -> Mux11/2
  Product/1 -> Mux11/1
  Mux/1 -> Scope3/1
  Mux13/1 -> Scope3/2
  Integrate and Dump/1 -> Product/1, Mux/1, Sign1/1
  GainOutMax/1 -> Scope9/2, Display9/1
  [RawData] -> Gain3/1
  Random Integer Generator1/1 -> Rate Transition1/1
  Rate Transition1/1 -> QPSK Modulator Baseband1/1
  Constant/1 -> NCO HDL Optimized/1
  NCO HDL Optimized/3 -> Terminator2/1
  Real Error Rate Calculation/1 -> Display16/1, Demux/1
  Complex to Real-Imag2/1 -> Integrate and Dump1/1
  Integrate and Dump2/1 -> Product1/1, Sign3/1, Mux13/1
  Integrate and Dump3/1 -> Product1/2, Sign2/1, Mux13/2
  Complex to Real-Imag2/2 -> Integrate and Dump3/1
  RealOut/1 -> Integrate and Dump/1, Real-Imag to Complex2/1
  Integrate and Dump1/1 -> Product/2, Mux/2, Sign/1
  Sign/1 -> Real Error Rate Calculation/1
  Sign1/1 -> Real Error Rate Calculation/2
  [Reset_n] -> LockImag/3(Rst_n), LockReal/3(Rst_n)
  Gain 20dB/V1/1 -> Bias1/1
  GainOutMax3/1 -> Gain4/1
  ReImPower/1(Power1) -> GainOutMax3/1
  AGC Ch1/1 -> RMS1/1, BER/1(In), Spectrum Analyzer/1, IntOffset Mixer/1, Delay9/1  "Ch1"
  Gain4/1 -> Scope6/1, Display1/1  "Sum"
  GainOutMax2/1 -> Gain7/1
  Gain7/1 -> Scope6/2, Display2/1  "Master"
  GainOutMax1/1 -> Gain8/1
  Gain8/1 -> Scope6/3, Display6/1  "Slave"
  ReImPower/3(Power3) -> GainOutMax1/1
  ReImPower/2(Power2) -> GainOutMax2/1
  Manual Switch5/1 -> ExtOffset Mixer/1, AWGN Channel1/1, [RawData]
  Constant21/1 -> Reset/1
  Gain3/1 -> Delay7/1
  Mux12/1 -> Scope3/4
  AddressSlice/1 -> Display8/1
  BER/1(Out1) -> Mux14/1
  AGC Ch2/1 -> BER1/1(In), RMS2/1, PhaseDetect/1, Spectrum Analyzer3/1, Complex to Real-Imag1/1  "Ch2"
  BER1/1(Out1) -> Mux14/2
  Mux16/1 -> Display11/1
  Mux14/1 -> Display14/1
  Mux15/1 -> Display13/1
  Lowpass Filter1/1 -> AGC Ch1/1  "Ch1"
  RMS2/1 -> Mux15/2
  RMS1/1 -> Mux15/1
  Step/1 -> Real Error Rate Calculation/3, Real Error Rate Calculation1/3, [RstStep]
  Mux11/1 -> Scope3/3
  AWGN Channel2/1 -> Gain6/1
  Gain6/1 -> Lowpass Filter2/1
  Lowpass Filter2/1 -> AGC Ch2/1  "Ch1"
  [RstStep] -> Display15/1
  OneMinusSlave/1 -> GainOutMax/1, Mult3/2, Mult2/2
  Sign2/1 -> Real Error Rate Calculation1/1
  Sign3/1 -> Real Error Rate Calculation1/2
  Real Error Rate Calculation1/1 -> Demux1/1, Display17/1
  Demux1/1 -> Mux16/2
  Demux/1 -> Mux16/1
  Address1/1 -> Display18/1
  Manual Switch1/1 -> Gain 20dB/V/1, AGCtoAWGN1/1(AGC)
  Gain 20dB/V/1 -> Bias/1
  AGCtoAWGN1/1(Variance) -> AWGN Channel1/2
  AGCtoAWGN2/1(Variance) -> AWGN Channel2/2
  AddSub1/1 -> AllZeros/1, AllOnes/1, GainOutMin/1, Mult5/2, Mult4/2, IIR_Out1/1, OneMinusSlave/2  "GainSlave"
  Constant3/1 -> OneMinusSlave/1
  LockReal1/1 -> LockThresh/1, Relational1/2, Relational/2
  Constant10/1 -> LockThreshold/1
  Constant15/1 -> LockHysterisis/1
  LockThreshold/1 -> LockReal1/1
  LockHysterisis/1 -> LockReal1/2
  Logical2/1 -> LockReal1/3, Locked/1, [Locked]
  LockThresh/1 -> Display19/1
  Delay9/1 -> Complex to Real-Imag/1
  Demux/2 -> Terminator3/1
  Demux/3 -> Terminator4/1
  Demux1/2 -> Terminator5/1
  Demux1/3 -> Terminator6/1
  LockReal/1(Out) -> RealLock/1, Relational/1
  Mux8/1 -> LockReal/1(In)
  IIR_Out1/1 -> Scope8/2  "SlaveGain"
  GainOutMin/1 -> Scope9/1, Display10/1  "Diff"
  IIR_Out5/1 -> Scope8/4  "Saturated"
  IIR_Out4/1 -> Scope8/3  "0Gt1"
  [Locks] -> Scope8/6  "Locks"
  IIR_Out2/1 -> Scope8/5  "Locked"
  Mult6/1 -> IIR_Out4/1, AddSub1/1
  Ch0AGC/1 -> IIR_Out6/1, DiffDB/1
  Ch1AGC/1 -> IIR_Out7/1, DiffDB/2
  Constant23/1 -> Manual Switch6/1
  Constant24/1 -> Manual Switch6/2
  Manual Switch6/1 -> Ch0GtCh1/1
  Constant26/1 -> Manual Switch4/1
  Constant25/1 -> Manual Switch4/2
  Manual Switch4/1 -> OverrideCh/1
  OverrideCh/1 -> Mux18/1
  Ch0GtCh1/1 -> Mux20/1
  Scale0/1 -> Ch0AGC/1
  Sum/1 -> Ch1AGC/1
  Scale1/1 -> Sum/1
  Constant17/1 -> Sum/2
  dB_Ratio/1 -> Mult1/1
  Divide/1 -> dB_Ratio/1
  High/1 -> Mux20/2
  High1/1 -> Mux20/3
  Mux20/1 -> Mux18/3
  DiffDB/1 -> Mux18/2
  Constant20/1 -> Divide/1
  [dB_Range] -> Divide/2
  Mult1/1 -> Slice/1, Address1/1, IIR_Out5/1, Current±3dB/1, IIR_Out/1
  Sign3dB/1 -> Delay8/1
  1.5dBHysteresis/1 -> Current±3dB/2
  Delay8/1 -> Inverter3/1, Current±3dB/3
  Inverter3/1 -> [Ch0GtCh1], AGC0_GT_AGC1/1
  Logical4/1 -> Delay8/3
  AGC0_GT_AGC1/1 -> Scope8/1, Display3/1  "Agc0GtAgc1"
  Current±3dB/1 -> Sign3dB/1
  Inverter2/1 -> Logical4/1
  [Locked] -> Inverter2/1
  AllOnes/1 -> Logical5/1
  AllZeros/1 -> Logical5/2
  [Reset] -> Delay8/2
  Constant22/1 -> [dB_Range], dB_Range/1
  Mux17/1 -> Scope8/8, Scope6/4, Mux12/2  "Gains"
  AGC1/1 -> Manual Switch1/1
  AGC2/1 -> Manual Switch3/1
  Manual Switch3/1 -> Gain 20dB/V1/1, AGCtoAWGN2/1(AGC)
  Logical5/1 -> Logical4/2, IIR_Out2/1
  Sine Wave3/1 -> Manual Switch3/2, Mux17/1
  Sine Wave1/1 -> Mux17/2, Manual Switch1/2
  IIR_Out/1 -> Scope4/1
  Mux18/1 -> IIR_Out3/1, Mult1/2
  IIR_Out3/1 -> Scope4/2
  IIR_Out7/1 -> Scope10/2
  IIR_Out6/1 -> Scope10/1
  Slice/1 -> AddressSlice/1, ROM/1
  ROM/1 -> Mult6/2
  dB_Offset/1 -> AddSub1/2
  dB_Range/1 -> Mult6/1
  PhaseSlide0/1(RealOut) -> Mult2/1, MaxRealOut/1, Real1Msb/1
  PhaseSlide0/2(ImagOut) -> Mult3/1, MaxImagOut/1, Imag1Msb/1
  PhaseSlide1/2(ImagOut) -> MinImagOut/1, Mult5/1, Imag2Msb/1
  PhaseSlide1/1(RealOut) -> Real2Msb/1, Mult4/1, MinRealOut/1
  Ch0Real/1 -> PhsDet1/3(SecRe), PhsDet0/1(PriRe)
  Ch0Imag/1 -> PhsDet1/4(SecIm), PhsDet0/2(PriIm)
  Ch1Real/1 -> PhsDet1/1(PriRe), PhsDet0/3(SecRe)
  Ch1Imag/1 -> PhsDet1/2(PriIm), PhsDet0/4(SecIm)
  Lag Coef/1 -> PhsDet1/7(LagCoef), PhsDet0/7(LagCoef)
  Lead Coef/1 -> PhsDet1/8(LeadCoef), PhsDet0/8(LeadCoef)
  SweepLmt/1 -> PhsDet1/5(Limit), PhsDet0/5(Limit)
  SwpRate/1 -> PhsDet1/6(SwpRate), PhsDet0/6(SwpRate)
  PhsDet0/1(OutARe) -> LagOutB7/1, Mux19/2
  PhsDet1/3(OutBRe) -> LagOutB2/1, Mux19/3
  PhsDet0/2(OutAIm) -> LagOutB5/1, Mux21/2
  PhsDet0/3(OutBRe) -> LagOutB6/1, Mux22/2
  PhsDet0/4(OutBIm) -> LagOutB8/1, Mux23/2
  PhsDet1/1(OutARe) -> LagOutB3/1, Mux22/3
  PhsDet0/6(Phase) -> PhaseSlide0/3(PhaseIn), PhaseA/1
  PhsDet0/5(LagOut) -> LagOutA/1
  PhsDet1/6(Phase) -> PhaseSlide1/3(PhaseIn), PhaseB/1
  PhsDet1/5(LagOut) -> LagOutB/1
  LagOutB/1 -> Mux3/2
  PhaseB/1 -> Mux2/2
  Reset/1 -> Inverter/1, [Reset]
  Inverter/1 -> [Reset_n]
  Mux1/1 -> Loop Filter Scope/1
  CW/1 -> Real-Imag to Complex3/2
  CW/2 -> Real-Imag to Complex3/1
  Constant1/1 -> CW/1
  CW/3 -> Terminator1/1
  QPSK Modulator Baseband1/1 -> Manual Switch5/1
  Real-Imag to Complex3/1 -> Manual Switch5/2
  PhsDet1/4(OutBIm) -> LagOutB4/1, Mux21/3
  PhsDet1/2(OutAIm) -> LagOutB1/1, Mux23/3
  Mux24/1 -> Scope11/1
  Mux25/1 -> Scope11/2
  Mux26/1 -> Scope11/3
  Mux27/1 -> Scope11/4
  LagOutB4/1 -> Mux27/2
  LagOutB1/1 -> Mux27/1
  LagOutB3/1 -> Mux26/1
  LagOutB2/1 -> Mux26/2
  LagOutB5/1 -> Mux25/1
  LagOutB6/1 -> Mux24/2
  LagOutB8/1 -> Mux25/2
  LagOutB7/1 -> Mux24/1
  Mux19/1 -> PhaseSlide0/1(Real)
  Mux21/1 -> PhaseSlide0/2(Imag)
  Mux22/1 -> PhaseSlide1/1(Real)
  Mux23/1 -> PhaseSlide1/2(Imag)
  [Ch0GtCh1] -> PhaseSlide0/4(ChSel), Inverter1/1, Mux23/1, Mux22/1, Mux21/1, Mux19/1
  Inverter1/1 -> PhaseSlide1/4(ChSel)
